simulink model "rotate_real"  (R2022a)
settings: Solver=FixedStepDiscrete  StartTime=0.0  StopTime=10  FixedStep=0.01  RelTol=1e-3  EnableMultiTasking=on
values from neighbouring files (symbols this model uses):
  axleLength = 0.136    [robotParameters.m]
  ticksPerRot = 20    [robotParameters.m]
  wheelR = 0.031    [robotParameters.m]
undefined symbols (not defined in the file or in its folder): InputPWM, WheelSpeed
libraries: arduinolib x8, mobileRoboticsTrainingLib x1
settings Model: ExtModeTrigDuration=2  Creator=heath  LastModifiedBy=heath
settings OptimizationCC: EnhancedBackFolding=on  PassReuseOutputArgsAs=Individual arguments  ZeroExternalMemoryAtStartup=off  ZeroInternalMemoryAtStartup=off  MaxStackSize=64  OptimizeBlockOrder=speed  DifferentSizesBufferReuse=on  OptimizationCustomize=off  EfficientTunableParamExpr=on
settings DebuggingCC: MultiTaskDSMMsg=none  ParameterTunabilityLossMsg=error
settings HardwareCC: ProdBitPerPointer=32  ProdBitPerSizeT=32  ProdBitPerPtrDiffT=32  ProdLargestAtomicInteger=Long  ProdLargestAtomicFloat=Double  ProdWordSize=32  ProdHWDeviceType=ARM Compatible->ARM Cortex  UseEmbeddedCoderFeatures=off  UseSimulinkCoderFeatures=off
settings SFSimCC: MATLABDynamicMemAlloc=off
settings RTWCC: SystemTargetFile=ert.tlc  HardwareBoard=Arduino Nano 33 IoT  TemplateMakefile=ert_default_tmf  Toolchain=Arduino ARM  BuildConfiguration=Faster Runs
settings CodeAppCC: ForceParamTrailComments=on  IgnoreCustomStorageClasses=off  OperatorAnnotations=on  SimulinkDataObjDesc=on  SFDataObjDesc=on  InsertBlockDesc=on
settings ERTTargetCC: SupportContinuousTime=on  SupportNonInlinedSFcns=on  SupportVariableSizeSignals=on  ExtModeTransport=3  ExtModeStaticAlloc=on  ExtModeStaticAllocSize=8192  ExtModeMexFile=ext_xcp  ExtModeIntrfLevel=Level2 - Open

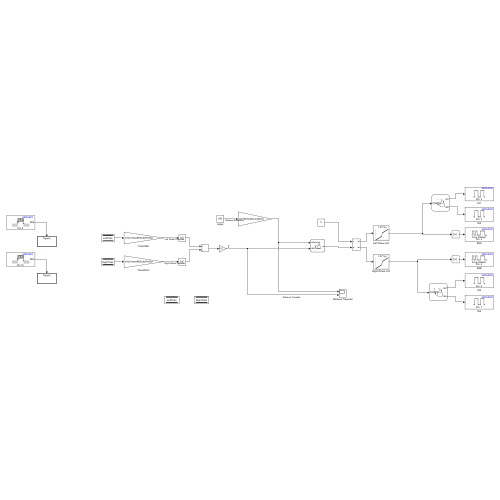
[thumbnail: Simulink's stored preview of the top-level diagram]
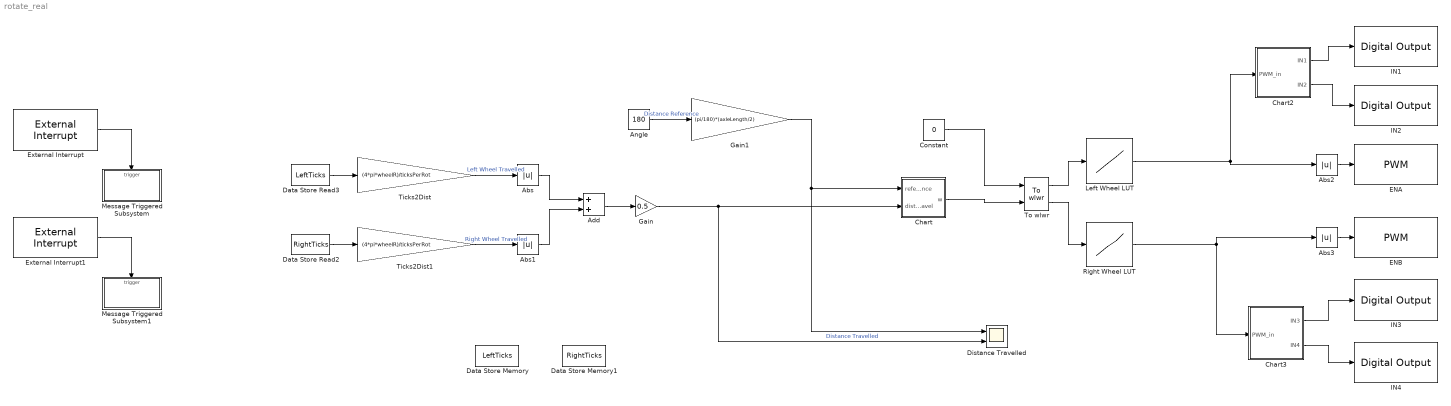
== system rotate_real ==
  Abs{,1..3} (4 alike) : Abs  SaturateOnIntegerOverflow=off
  Add : Sum
  Angle : Constant  Value=180
  Chart : Stateflow chart  TreatAsAtomicUnit=on
  Chart2 : Stateflow chart  TreatAsAtomicUnit=on
  Chart3 : Stateflow chart  TreatAsAtomicUnit=on
  Constant : Constant  Value=0
  Data Store Memory : DataStoreMemory  DataStoreName=LeftTicks  WriteAfterWriteMsg=warning  ShowAdditionalParam=off
  Data Store Memory1 : DataStoreMemory  DataStoreName=RightTicks  WriteAfterWriteMsg=warning  ShowAdditionalParam=off
  Data Store Read2 : DataStoreRead  DataStoreName=RightTicks  IndexOptions=Index vector (dialog)  Indices=1  OutputSizes=1
  Data Store Read3 : DataStoreRead  DataStoreName=LeftTicks  IndexOptions=Index vector (dialog)  Indices=1  OutputSizes=1
  Distance Travelled : Scope  NumInputPorts=2
  ENA : arduinolib/PWM  pinNumber=3  frequencyType=Default  desiredFrequency=490.2  achievableFrequency=490.2
  ENB : arduinolib/PWM  pinNumber=2  frequencyType=Default  desiredFrequency=490.2  achievableFrequency=490.2
  External Interrupt : arduinolib/External Interrupt  Pin=9  PullUp=off  Mode=RISING  InterruptSimulationInput=off
      settings: SourceProductBaseCode=ARDUINO
  External Interrupt1 : arduinolib/External Interrupt  Pin=10  PullUp=off  Mode=RISING  InterruptSimulationInput=off
      settings: SourceProductBaseCode=ARDUINO
  Gain : Gain  Gain=0.5
  Gain1 : Gain  Gain=(pi/180)*(axleLength/2)
  IN1 : arduinolib/Digital Output  pinNumber=4  Direction=output  blockPlatform=arduino
  IN2 : arduinolib/Digital Output  pinNumber=5  Direction=output  blockPlatform=arduino
  IN3 : arduinolib/Digital Output  pinNumber=6  Direction=output  blockPlatform=arduino
  IN4 : arduinolib/Digital Output  pinNumber=7  Direction=output  blockPlatform=arduino
  Left Wheel LUT : Lookup_n-D  NumberOfTableDimensions=1  BreakpointsForDimension1=WheelSpeed  Table=InputPWM  InternalRulePriority=Speed  RndMeth=Simplest
  Message Triggered Subsystem : Subsystem  TreatAsAtomicUnit=on
  Message Triggered Subsystem1 : Subsystem  TreatAsAtomicUnit=on
  Right Wheel LUT : Lookup_n-D  NumberOfTableDimensions=1  BreakpointsForDimension1=WheelSpeed  Table=InputPWM  InternalRulePriority=Speed  RndMeth=Simplest
  Ticks2Dist : Gain  Gain=(4*pi*wheelR)/ticksPerRot
  Ticks2Dist1 : Gain  Gain=(4*pi*wheelR)/ticksPerRot
  To wlwr : mobileRoboticsTrainingLib/To wlwr  axleLength=axleLength  wheelR=wheelR
  wires:
  Ticks2Dist/1 -> Abs/1  "Left Wheel Travelled"
  Ticks2Dist1/1 -> Abs1/1  "Right Wheel Travelled"
  Add/1 -> Gain/1
  Gain/1 -> Distance Travelled/2, Chart/2(distTravel)  "Distance Travelled"
  To wlwr/1 -> Left Wheel LUT/1
  To wlwr/2 -> Right Wheel LUT/1
  Angle/1 -> Gain1/1  "Distance Reference"
  Abs/1 -> Add/1
  Abs1/1 -> Add/2
  Constant/1 -> To wlwr/1
  Gain1/1 -> Distance Travelled/1, Chart/1(reference)
  Chart3/1(IN3) -> IN3/1
  Chart2/1(IN1) -> IN1/1
  Chart2/2(IN2) -> IN2/1
  Abs2/1 -> ENA/1
  Left Wheel LUT/1 -> Abs2/1, Chart2/1(PWM_in)
  Abs3/1 -> ENB/1
  Chart3/2(IN4) -> IN4/1
  Right Wheel LUT/1 -> Abs3/1, Chart3/1(PWM_in)
  External Interrupt/1 -> Message Triggered Subsystem/Trigger
  Data Store Read2/1 -> Ticks2Dist1/1
  External Interrupt1/1 -> Message Triggered Subsystem1/Trigger
  Data Store Read3/1 -> Ticks2Dist/1
  Chart/1(w) -> To wlwr/2

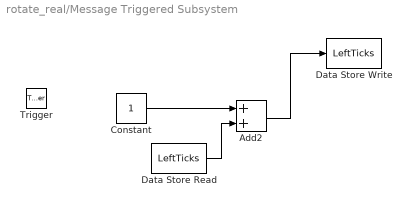
== system rotate_real/Message Triggered Subsystem ==
  Trigger : TriggerPort  TriggerType=function-call  VariantControl=(inherit)  PortDimensions=1
  Add2 : Sum
  Constant : Constant
  Data Store Read : DataStoreRead  DataStoreName=LeftTicks  IndexOptions=Index vector (dialog)  Indices=1  OutputSizes=1
  Data Store Write : DataStoreWrite  DataStoreName=LeftTicks  IndexOptions=Index vector (dialog)  Indices=1  OutputSizes=1
  wires:
  Add2/1 -> Data Store Write/1
  Constant/1 -> Add2/1
  Data Store Read/1 -> Add2/2

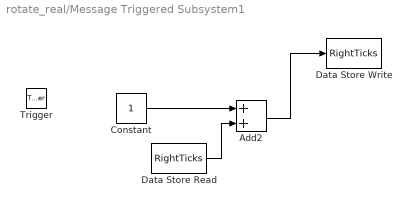
== system rotate_real/Message Triggered Subsystem1 ==
  Trigger : TriggerPort  TriggerType=function-call  VariantControl=(inherit)  PortDimensions=1
  Add2 : Sum
  Constant : Constant
  Data Store Read : DataStoreRead  DataStoreName=RightTicks  IndexOptions=Index vector (dialog)  Indices=1  OutputSizes=1
  Data Store Write : DataStoreWrite  DataStoreName=RightTicks  IndexOptions=Index vector (dialog)  Indices=1  OutputSizes=1
  wires:
  Add2/1 -> Data Store Write/1
  Constant/1 -> Add2/1
  Data Store Read/1 -> Add2/2

== stateflow chart rotate_real/Chart2 ==
  state Forward
    entry:
    IN1 = 1;
    IN2 = 0;
  state Back
    entry:
    IN1 = 0;
    IN2 = 1;
  (default) -> Forward
  Forward -> Back : [PWM_in<0]
  Back -> Forward : [PWM_in>=0]
  data: PWM_in input; IN1 output; IN2 output

== stateflow chart rotate_real/Chart ==
  state MoveForward
    entry:
    w = 2;
  state Stop
    entry:
    w = 0;
  (default) -> MoveForward
  MoveForward -> Stop : [distTravel > reference]
  data: reference input; distTravel input; w output

== stateflow chart rotate_real/Chart3 ==
  state Forward
    entry:
    IN4 = 0;
    IN3 = 1;
  state Back
    entry:
    IN4 = 1;
    IN3 = 0;
  (default) -> Forward
  Forward -> Back : [PWM_in<0]
  Back -> Forward : [PWM_in>=0]
  data: PWM_in input; IN3 output; IN4 output
